simulink model "ANC_Prototype"  (R2013a)
settings: Solver=VariableStepDiscrete  StartTime=0.0  StopTime=20  MaxStep=0.1  RelTol=1e-3
libraries: dspadpt3 x1, commnoisgen2 x1
settings Model: Creator=sebin  LastModifiedBy=sebin

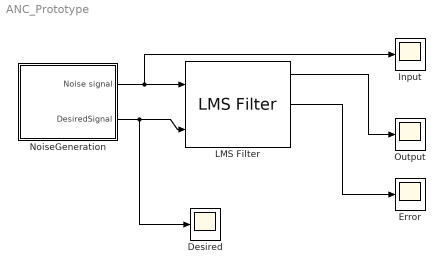
== system ANC_Prototype ==
  Desired : Scope
      settings: SaveName=ScopeData3
  Error : Scope
  "Input " : Scope
      settings: SaveName=ScopeData2
  LMS Filter : dspadpt3/LMS Filter  Algo=LMS  L=32  stepflag=Dialog  mu=0.01  leakage=1.0  ic=0  Adapt=off  resetflag=None  weights=on  secondCoeffMode=User-defined  secondCoeffWordLength=2  secondCoeffFracLength=15  accum2Mode=User-defined  accum2FracLength=20  prodOutput2Mode=User-defined  prodOutput2FracLength=20  prodOutput3Mode=User-defined  prodOutput3FracLength=20  prodOutput4Mode=User-defined  prodOutput4FracLength=20  quotientMode=User-defined  quotientFracLength=20  roundingMode=Floor  overflowMode=off  addnparflag=off
  NoiseGeneration : Subsystem
  Output : Scope
  wires:
  NoiseGeneration/1(Noise signal) -> "Input "/1, LMS Filter/1
  NoiseGeneration/2("DesiredSignal ") -> Desired/1, LMS Filter/2
  LMS Filter/1 -> Output/1
  LMS Filter/2 -> Error/1

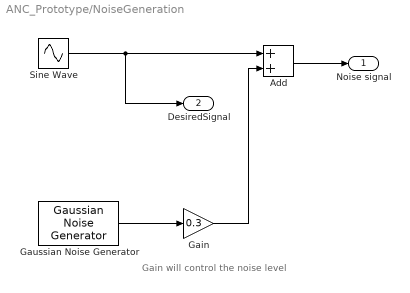
== system ANC_Prototype/NoiseGeneration ==
  note: Gain will control the noise level
  Add : Sum
  Gain : Gain  Gain=0.3
  Gaussian Noise Generator : commnoisgen2/Gaussian Noise Generator  m=0  d=1  s=41  Ts=1  frameBased=off  sampPerFrame=1  orient=off  outDataType=double
  Sine Wave : Sin  SampleTime=0
  Noise signal : Outport
  "DesiredSignal " : Outport  Port=2
  wires:
  Sine Wave/1 -> "DesiredSignal "/1, Add/1
  Gaussian Noise Generator/1 -> Gain/1
  Gain/1 -> Add/2
  Add/1 -> Noise signal/1
